simulink model "fxio_uart_receive_isr_s32k11x"  (Simulink 9.0)
settings: Solver=FixedStepDiscrete  StartTime=0.0  StopTime=10.0  FixedStep=0.1  RelTol=1e-3
InitFcn:
  | mbd_s32k_consistency_checks(bdroot(gcs));
undefined symbols (not defined in the file): LQFP, thumb
libraries: mbd_s32k1xx_ec_toolbox x5, simulink x1
Description:
  | This demo shows how to configure the S32K118EVB to receive data over UART (emulation via FlexIO).
  | 
  | This example requires another board running the fxio_uart_transmit_isr_s32k11x model.
  | 
  | HW prerequisite:
  | - 2x S32K118EVB
  | - Connect:
  | PTD0 (FXIO_UART_Tx from the other board) - PTD1 (FXIO_UART_Rx from this board)
  | 
  | Verification:
  | - Each time a character is received the red LED toggles
  | - Open the FreeMASTER project associated with this example, and check if the data iterates through [0,7] interval.
settings Model: Creator=NXP MBDT Team  LastModifiedBy=nxf35172
settings DataIOCC: ExternalInput=off  InitialState=off  SaveFormat=Dataset  SaveOutput=off  SignalLogging=off  SaveTime=off
settings OptimizationCC: DefaultParameterBehavior=Inlined  EnhancedBackFolding=on  PassReuseOutputArgsAs=Individual arguments  LifeSpan=auto
settings DebuggingCC: UnderspecifiedInitializationDetection=Simplified  MergeDetectMultiDrivingBlocksExec=error  InheritedTsInSrcMsg=none  SingleTaskRateTransMsg=error  ParameterTunabilityLossMsg=error  UnconnectedInputMsg=error  UnconnectedOutputMsg=error  UnconnectedLineMsg=error  UnknownTsInhSupMsg=error  SFUnexpectedBacktrackingDiag=error  SFNoUnconditionalDefaultTransitionDiag=error  SFExecutionAtInitializationDiag=warning
settings HardwareCC: ProdLargestAtomicInteger=Long  ProdLargestAtomicFloat=Double  ProdIntDivRoundTo=Zero  ProdEndianess=LittleEndian  ProdHWDeviceType=ARM Compatible->ARM Cortex
settings ModelReferenceCC: PropagateSignalLabelsOutOfModel=on
settings SFSimCC: MATLABDynamicMemAlloc=off
settings RTWCC: SystemTargetFile=mbd_s32k.tlc  MakeCommand=mbd_s32k_make_rtw COPY_MDLREF_INCLUDES=0  TemplateMakefile=mbd_s32k.tmf  Description=Model Based Design Toolbox S32K14x Code Generation Target  GenerateReport=on  IncludeHyperlinkInReport=on  LaunchReport=on  GenerateTraceInfo=on  GenerateTraceReport=on  GenerateTraceReportSl=on  GenerateTraceReportSf=on  GenerateTraceReportEml=on
settings CodeAppCC: ForceParamTrailComments=on  IgnoreCustomStorageClasses=off  OperatorAnnotations=on  SimulinkDataObjDesc=on  SFDataObjDesc=on  InsertBlockDesc=on
settings STFCustomTargetCC: TargetLangStandard=C99 (ISO)  MultiwordLength=256  CombineOutputUpdateFcns=on  ERTCustomFileBanners=on  SupportContinuousTime=off  SupportNonInlinedSFcns=off  RemoveResetFunc=on  MATLABClassNameForMDSCustomization=Simulink.SoftwareTarget.ERTCustomization  GRTInterface=off  SystemTargetFile=mbd_s32k14.tlc
settings ERTTargetCC: TargetLangStandard=C99 (ISO)  ParMdlRefBuildCompliant=off  CompOptLevelCompliant=off  ConcurrentExecutionCompliant=off  ModelStepFunctionPrototypeControlCompliant=off  CPPClassGenCompliant=off  UseToolchainInfoCompliant=off  InlinedParameterPlacement=NonHierarchical  ERTSrcFileBannerTemplate=mbd_ert_code_template.cgt  ERTHdrFileBannerTemplate=mbd_ert_code_template.cgt  ERTDataSrcFileTemplate=mbd_ert_code_template.cgt  ERTDataHdrFileTemplate=mbd_ert_code_template.cgt  ERTCustomFileTemplate=example_file_process.tlc
settings ConfigComp: CovMetricSettings=dwe  CovHtmlReporting=off  CovSaveCumulativeToWorkspaceVar=off  CovSaveSingleToWorkspaceVar=off  CovExternalEMLEnable=on

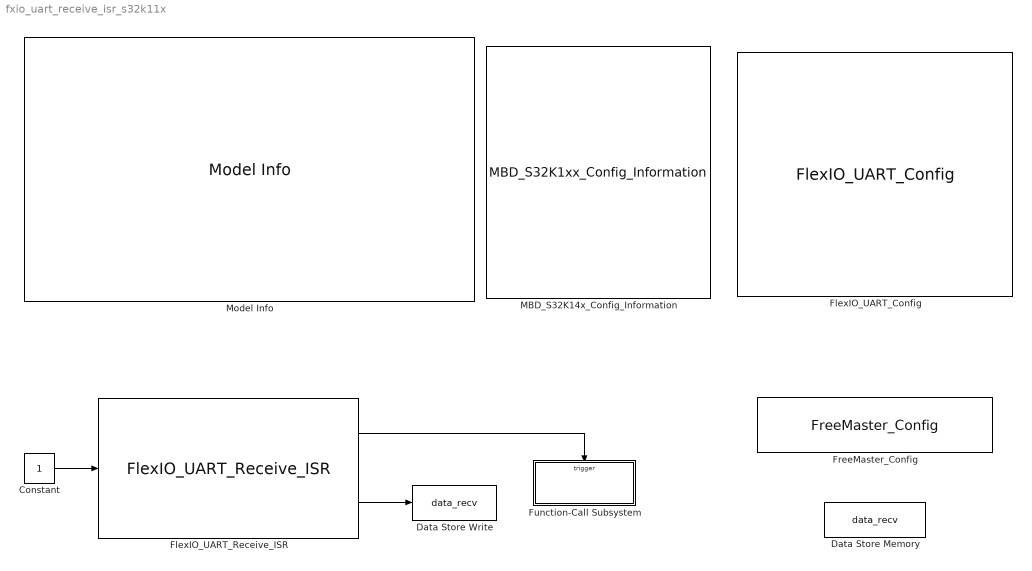
== system fxio_uart_receive_isr_s32k11x ==
  Constant : Constant  OutDataTypeStr=uint32
  Data Store Memory : DataStoreMemory  DataStoreName=data_recv  ReadBeforeWriteMsg=warning  WriteAfterWriteMsg=warning  WriteAfterReadMsg=warning  ShowAdditionalParam=off
  Data Store Write : DataStoreWrite  DataStoreName=data_recv
  "FlexIO_UART_Config " : mbd_s32k1xx_ec_toolbox/Communication Blocks/FlexIO Blocks /FlexIO UART Blocks/FlexIO_UART_Config   Priority=1  InstanceNumber=0  DriverType=Interrupts  BitCount=8  BaudRate=115200  TxPin=PTD0: [FXIO_D0 | FlexIO Bi-directional Shift/timer I/O]  RxPin=PTD1: [FXIO_D1 | FlexIO Bi-directional Shift/timer I/O]
  FlexIO_UART_Receive_ISR : mbd_s32k1xx_ec_toolbox/Communication Blocks/FlexIO Blocks /FlexIO UART Blocks/FlexIO_UART_Receive_ISR  Priority=1  InstanceNumber=0
  FreeMaster_Config : mbd_s32k1xx_ec_toolbox/Utility Blocks/FreeMaster_Config  interface=LPUART0  baudrate=115200  rxd=PTB0: [LPUART0_RX | Receive]  txd=PTB1: [LPUART0_TX | Transmit]  mode=Short Interrupt  isr_prio=2  show_adv_opts=on  use_scope=on  max_scope_vars=8  use_recorder=on  max_rec_vars=8  rec_buff_size=1024  rec_timebase=0 seconds  comm_buffer_size_auto=on  comm_buffer_size=255  comm_rqueue_size_default=on  comm_rqueue_size=32
  Function-Call Subsystem : Subsystem  TreatAsAtomicUnit=on
  MBD_S32K14x_Config_Information : mbd_s32k1xx_ec_toolbox/MBD_S32K1xx_Config_Information  Priority=0  mbdt_ver=0  disp_str=|  config_params=[]  mcu_target_name=S32K118  mcu_target_package=64-LQFP  mcu_target_sram_size=25KB  mcu_system_clock_freq=40  mcu_xtal_freq=External 40  mcu_steptick_timer=LPIT Channel 0  mcu_steptick_prio=0  ds_import_enable=on  target_compiler=GCC  target_memory=FLASH  gcc_target_compile_opts=-mcpu=cortex-m0plus -mthumb -O1 -g -gstrict-dwarf  gcc_target_assemble_opts=-mcpu=cortex-m0plus -mthumb -g  gcc_target_link_opts=-mcpu=cortex-m0plus -mthumb  gcc_target_default_lcf=on  gcc_target_user_lcf=S32K118_25_flash.ld  ghs_target_compile_opts=-mcpu=cortexm0plus -mthumb -fsoft -Ogeneral -Wundef -Wimplicit-int -Wshadow -Wtrigraphs --no_commons --gnu_asm -gnu99 -gdwarf-2 -G  ghs_target_assemble_opts=-mcpu=cortexm0plus -mthumb -fsoft --gnu_asm  ghs_target_link_opts=-mcpu=cortexm0plus -mthumb -fsoft  ghs_target_default_lcf=off  ghs_target_user_lcf=S32K118_25_flash.ld  iar_target_compile_opts=--thumb -Ol -e --debug --dlib_config normal  iar_target_assemble_opts=--thumb  iar_target_link_opts=--no_exceptions --vfe --inline  iar_target_default_lcf=off  iar_target_user_lcf=S32K118_25_flash.icf  pil_download_enable=off  rbl_download_enable=on  rbl_start_delay=5000000  rbl_download_interface=OpenSDA  rbl_restart_request=off  rbl_com_port=Custom  rbl_com_port_custom=COM1  pil_download_rate=57600  pil_opensda_drive=Custom  pil_opensda_drive_custom=D  pil_uart_instance=0  pil_uart_rx=PTB0: [LPUART0_RX | Receive]  pil_uart_tx=PTB1: [LPUART0_TX | Transmit]  FTM_PWM_PcrCheckEnDis=on  FTM_Input_Edge_Inputs_PcrCheckEnDis=on  FTM_Dual_Edge_Inputs_PcrCheckEnDis=on  FTM_Quadrature_Inputs_PcrCheckEnDis=on  FTM_Hall_Sensor_Inputs_PcrCheckEnDis=on  LPTMR_PcrCheckEnDis=on  PIT_PcrCheckEnDis=on  RTC_PcrCheckEnDis=on  FlexCAN_PcrCheckEnDis=on  LIN_PcrCheckEnDis=on  FlexIO_PcrCheckEnDis=on  LPI2C_PcrCheckEnDis=on  LPSPI_PcrCheckEnDis=on  LPUART_PcrCheckEnDis=on  CMP_PcrCheckEnDis=on  GPIO_OutputPcrCheckEnDis=on  GPIO_InputPcrCheckEnDis=on  SBC_PcrCheckEnDis=on  AMMCLIB_PcrCheckEnDis=on  FM_PcrCheckEnDis=on  Profile_PcrCheckEnDis=on  ConfigParams_PcrCheckEnDis=on  ModelRef_PcrCheckEnDis=on  PDB0_PcrCheckEnDis=on  CSEc_PcrCheckEnDis=on  eDMA_PcrCheckEnDis=on  ADC_PcrCheckEnDis=on  WDOG_PcrCheckEnDis=on
      | Target : S32K144-64KB_SRAM
      | Package : 100-pin
      | System clock : 80 MHz
      | XTAL clock : External 8 MHz
      | Compiler : GCC
      | Target Type : FLASH
      | Download Code after build : (OpenSDA: D)
      | Step Tick Interrupt Priority : 15
  Model Info : simulink/Model-Wide Utilities/Model Info  Frame=off  DisplayStringWithTags=|  HorizontalTextAlignment=Left  LeftAlignmentValue=0.02
      | Model Name: %<ModelName>
      | 
      | Description: %<Description>
  wires:
  Constant/1 -> FlexIO_UART_Receive_ISR/1
  FlexIO_UART_Receive_ISR/2 -> Data Store Write/1
  FlexIO_UART_Receive_ISR/1 -> Function-Call Subsystem/Trigger

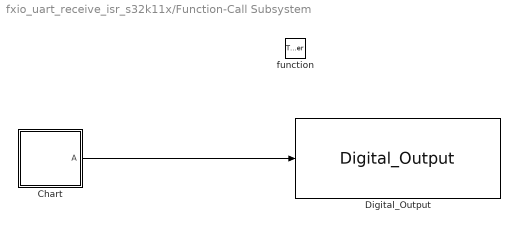
== system fxio_uart_receive_isr_s32k11x/Function-Call Subsystem ==
  function : TriggerPort  TriggerType=function-call  VariantControl=Variant
  Chart : Stateflow chart  TreatAsAtomicUnit=on
  Digital_Output : mbd_s32k1xx_ec_toolbox/GPIO Blocks/Digital_Output  gpio_pin=PTD16: [PTD16 | Port D I/O]  init_val=Low  drive_strength=Low
  wires:
  Chart/1(" A") -> Digital_Output/1

== stateflow chart Function-Call Subsystem/Chart ==
  state A
  state A1
  (default) -> A
  A -> A1
  A1 -> A
  data: A output boolean [0..1]
